simulink library "xrbsComm_r4"  (Simulink 7.1)
PreLoadFcn:
  | warning('off','MATLAB:mex:deprecatedExtension');xlmeta;com.xilinx.sysgen.util.StrategyUtil.loadAllStrategyNames();
undefined symbols (not defined in the file or in its folder): calc_path_data, gcbh, mfcm_matrix_rom, oct2dec, xlBlockLoadCallback
libraries: xbsIndex_r4 x851, mfcm_block_lib_v1 x5, xrbsComm_r4 x1, mfcm_misc_lib_v1 x1
(part 5 of 8)

== system xrbsComm_r4/White Gaussian  Noise Generator/Box-Muller2/fr1/lfsr_41_2/x6 ==
  " " : Inport  OutDataType=sfix(16)  OutScaling=2^0
  reset : Inport  Port=2  OutDataType=sfix(16)  OutScaling=2^0
  ASR : Subsystem  mask{init=[init(8) init(7) init(6) init(5) init(4) init(3) init(2) init(1)]}
      mask prompts: init "Initial Value"
      mask init:
      | init_size = size(init);
      | asr_length = init_size(2);
  Register1 : xbsIndex_r4/Register  init=init(9)  rst=on  en=off  dbl_ovrd=off  block_type=register
      settings: xl_area=[0, 0, 0, 0, 0, 0, 0]  block_version=VER_STRING_GOES_HERE
  z-9 : Outport  OutDataType=sfix(16)  OutScaling=2^0
  wires:
  ASR/1(dout) -> z-9/1
  " "/1 -> Register1/1
  Register1/1 -> ASR/1(din)
  reset/1 -> Register1/2

== system xrbsComm_r4/White Gaussian  Noise Generator/Box-Muller2/fr1/lfsr_41_2/x7 ==
  " " : Inport  OutDataType=sfix(16)  OutScaling=2^0
  reset : Inport  Port=2  OutDataType=sfix(16)  OutScaling=2^0
  ASR : Subsystem  mask{init=[init(8) init(7) init(6) init(5) init(4) init(3) init(2) init(1)]}
      mask prompts: init "Initial Value"
      mask init:
      | init_size = size(init);
      | asr_length = init_size(2);
  Register1 : xbsIndex_r4/Register  init=init(9)  rst=on  en=off  dbl_ovrd=off  block_type=register
      settings: xl_area=[0, 0, 0, 0, 0, 0, 0]  block_version=VER_STRING_GOES_HERE
  z-9 : Outport  OutDataType=sfix(16)  OutScaling=2^0
  wires:
  ASR/1(dout) -> z-9/1
  Register1/1 -> ASR/1(din)
  " "/1 -> Register1/1
  reset/1 -> Register1/2

== system xrbsComm_r4/White Gaussian  Noise Generator/Box-Muller2/g2/lfsr_47_5/x10 ==
  "  " : Inport  OutDataType=sfix(16)  OutScaling=2^0
  reset : Inport  Port=2  OutDataType=sfix(16)  OutScaling=2^0
  ASR : Subsystem  mask{init=[init(4) init(3) init(2) init(1)]}
      mask prompts: init "Initial Value"
      mask init:
      | init_size = size(init);
      | asr_length = init_size(2);
  Register5 : xbsIndex_r4/Register  init=init(5)  rst=on  en=off  dbl_ovrd=off  block_type=register
      settings: xl_area=[0, 0, 0, 0, 0, 0, 0]  block_version=VER_STRING_GOES_HERE
  z-5 : Outport  OutDataType=sfix(16)  OutScaling=2^0
  wires:
  ASR/1(dout) -> z-5/1
  Register5/1 -> ASR/1(din)
  "  "/1 -> Register5/1
  reset/1 -> Register5/2

== system xrbsComm_r4/White Gaussian  Noise Generator/Box-Muller2/g2/lfsr_47_5/x11 ==
  " " : Inport  OutDataType=sfix(16)  OutScaling=2^0
  reset : Inport  Port=2  OutDataType=sfix(16)  OutScaling=2^0
  ASR : Subsystem  mask{init=[init(4) init(3) init(2) init(1)]}
      mask prompts: init "Initial Value"
      mask init:
      | init_size = size(init);
      | asr_length = init_size(2);
  Register : xbsIndex_r4/Register  init=init(5)  rst=on  en=off  dbl_ovrd=off  block_type=register
      settings: xl_area=[0, 0, 0, 0, 0, 0, 0]  block_version=VER_STRING_GOES_HERE
  z-5 : Outport  OutDataType=sfix(16)  OutScaling=2^0
  wires:
  ASR/1(dout) -> z-5/1
  Register/1 -> ASR/1(din)
  " "/1 -> Register/1
  reset/1 -> Register/2

== system xrbsComm_r4/White Gaussian  Noise Generator/Box-Muller2/g2/lfsr_47_5/x12 ==
  " " : Inport  OutDataType=sfix(16)  OutScaling=2^0
  reset : Inport  Port=2  OutDataType=sfix(16)  OutScaling=2^0
  ASR : Subsystem  mask{init=[init(4) init(3) init(2) init(1)]}
      mask prompts: init "Initial Value"
      mask init:
      | init_size = size(init);
      | asr_length = init_size(2);
  Register : xbsIndex_r4/Register  init=init(5)  rst=on  en=off  dbl_ovrd=off  block_type=register
      settings: xl_area=[0, 0, 0, 0, 0, 0, 0]  block_version=VER_STRING_GOES_HERE
  z-5 : Outport  OutDataType=sfix(16)  OutScaling=2^0
  wires:
  ASR/1(dout) -> z-5/1
  Register/1 -> ASR/1(din)
  " "/1 -> Register/1
  reset/1 -> Register/2

== system xrbsComm_r4/White Gaussian  Noise Generator/Box-Muller2/g2/lfsr_47_5/x13 ==
  note: reset
  " " : Inport  OutDataType=sfix(16)  OutScaling=2^0
  " 1" : Inport  Port=2  OutDataType=sfix(16)  OutScaling=2^0
  ASR : Subsystem  mask{init=[init(4) init(3) init(2) init(1)]}
      mask prompts: init "Initial Value"
      mask init:
      | init_size = size(init);
      | asr_length = init_size(2);
  Register : xbsIndex_r4/Register  init=init(5)  rst=on  en=off  dbl_ovrd=off  block_type=register
      settings: xl_area=[0, 0, 0, 0, 0, 0, 0]  block_version=VER_STRING_GOES_HERE
  z-5 : Outport  OutDataType=sfix(16)  OutScaling=2^0
  wires:
  ASR/1(dout) -> z-5/1
  Register/1 -> ASR/1(din)
  " "/1 -> Register/1
  " 1"/1 -> Register/2

== system xrbsComm_r4/White Gaussian  Noise Generator/Box-Muller2/g2/lfsr_47_5/x14 ==
  " " : Inport  OutDataType=sfix(16)  OutScaling=2^0
  reset : Inport  Port=2  OutDataType=sfix(16)  OutScaling=2^0
  ASR : Subsystem  mask{init=[init(4) init(3) init(2) init(1)]}
      mask prompts: init "Initial Value"
      mask init:
      | init_size = size(init);
      | asr_length = init_size(2);
  Register : xbsIndex_r4/Register  init=init(5)  rst=on  en=off  dbl_ovrd=off  block_type=register
      settings: xl_area=[0, 0, 0, 0, 0, 0, 0]  block_version=VER_STRING_GOES_HERE
  z-5 : Outport  OutDataType=sfix(16)  OutScaling=2^0
  wires:
  ASR/1(dout) -> z-5/1
  Register/1 -> ASR/1(din)
  " "/1 -> Register/1
  reset/1 -> Register/2

== system xrbsComm_r4/White Gaussian  Noise Generator/Box-Muller2/g2/lfsr_47_5/x15 ==
  " " : Inport  OutDataType=sfix(16)  OutScaling=2^0
  reset : Inport  Port=2  OutDataType=sfix(16)  OutScaling=2^0
  ASR : Subsystem  mask{init=[init(4) init(3) init(2) init(1)]}
      mask prompts: init "Initial Value"
      mask init:
      | init_size = size(init);
      | asr_length = init_size(2);
  Register : xbsIndex_r4/Register  init=init(5)  rst=on  en=off  dbl_ovrd=off  block_type=register
      settings: xl_area=[0, 0, 0, 0, 0, 0, 0]  block_version=VER_STRING_GOES_HERE
  z-5 : Outport  OutDataType=sfix(16)  OutScaling=2^0
  wires:
  ASR/1(dout) -> z-5/1
  Register/1 -> ASR/1(din)
  " "/1 -> Register/1
  reset/1 -> Register/2

== system xrbsComm_r4/White Gaussian  Noise Generator/Box-Muller2/g2/lfsr_47_5/x16 ==
  " " : Inport  OutDataType=sfix(16)  OutScaling=2^0
  reset : Inport  Port=2  OutDataType=sfix(16)  OutScaling=2^0
  ASR : Subsystem  mask{init=[init(3) init(2) init(1)]}
      mask prompts: init "Initial Value"
      mask init:
      | init_size = size(init);
      | asr_length = init_size(2);
  Register : xbsIndex_r4/Register  init=init(4)  rst=on  en=off  dbl_ovrd=off  block_type=register
      settings: xl_area=[0, 0, 0, 0, 0, 0, 0]  block_version=VER_STRING_GOES_HERE
  z-4 : Outport  OutDataType=sfix(16)  OutScaling=2^0
  wires:
  ASR/1(dout) -> z-4/1
  Register/1 -> ASR/1(din)
  " "/1 -> Register/1
  reset/1 -> Register/2

== system xrbsComm_r4/White Gaussian  Noise Generator/Box-Muller2/g2/lfsr_47_5/x9 ==
  " " : Inport  OutDataType=sfix(16)  OutScaling=2^0
  reset : Inport  Port=2  OutDataType=sfix(16)  OutScaling=2^0
  ASR : Subsystem  mask{init=[init(4) init(3) init(2) init(1)]}
      mask prompts: init "Initial Value"
      mask init:
      | init_size = size(init);
      | asr_length = init_size(2);
  Register : xbsIndex_r4/Register  init=init(5)  rst=on  en=off  dbl_ovrd=off  block_type=register
      settings: xl_area=[0, 0, 0, 0, 0, 0, 0]  block_version=VER_STRING_GOES_HERE
  z-5 : Outport  OutDataType=sfix(16)  OutScaling=2^0
  wires:
  ASR/1(dout) -> z-5/1
  Register/1 -> ASR/1(din)
  " "/1 -> Register/1
  reset/1 -> Register/2

== system xrbsComm_r4/White Gaussian  Noise Generator/Box-Muller3/fr1/lfsr_17_2/x1 ==
  " " : Inport  OutDataType=sfix(16)  OutScaling=2^0
  " reset" : Inport  Port=2  OutDataType=sfix(16)  OutScaling=2^0
  ASR : Subsystem  mask{init=[init(2) init(1)]}
      mask prompts: init "Initial Value"
      mask init:
      | init_size = size(init);
      | asr_length = init_size(2);
  Register4 : xbsIndex_r4/Register  init=init(3)  rst=on  en=off  dbl_ovrd=off  block_type=register
      settings: xl_area=[0, 0, 0, 0, 0, 0, 0]  block_version=VER_STRING_GOES_HERE
  z-3 : Outport  OutDataType=sfix(16)  OutScaling=2^0
  wires:
  " "/1 -> Register4/1
  ASR/1(dout) -> z-3/1
  Register4/1 -> ASR/1(din)
  " reset"/1 -> Register4/2

== system xrbsComm_r4/White Gaussian  Noise Generator/Box-Muller3/fr1/lfsr_17_2/x5 ==
  " " : Inport  OutDataType=sfix(16)  OutScaling=2^0
  reset : Inport  Port=2  OutDataType=sfix(16)  OutScaling=2^0
  ASR : Subsystem  mask{init=[init(3) init(2) init(1)]}
      mask prompts: init "Initial Value"
      mask init:
      | init_size = size(init);
      | asr_length = init_size(2);
  Register5 : xbsIndex_r4/Register  init=init(4)  rst=on  en=off  dbl_ovrd=off  block_type=register
      settings: xl_area=[0, 0, 0, 0, 0, 0, 0]  block_version=VER_STRING_GOES_HERE
  z-4 : Outport  OutDataType=sfix(16)  OutScaling=2^0
  wires:
  ASR/1(dout) -> z-4/1
  Register5/1 -> ASR/1(din)
  " "/1 -> Register5/1
  reset/1 -> Register5/2

== system xrbsComm_r4/White Gaussian  Noise Generator/Box-Muller3/fr1/lfsr_17_2/x6 ==
  " " : Inport  OutDataType=sfix(16)  OutScaling=2^0
  " reset" : Inport  Port=2  OutDataType=sfix(16)  OutScaling=2^0
  ASR : Subsystem  mask{init=[init(2) init(1)]}
      mask prompts: init "Initial Value"
      mask init:
      | init_size = size(init);
      | asr_length = init_size(2);
  Register4 : xbsIndex_r4/Register  init=init(3)  rst=on  en=off  dbl_ovrd=off  block_type=register
      settings: xl_area=[0, 0, 0, 0, 0, 0, 0]  block_version=VER_STRING_GOES_HERE
  z-3 : Outport  OutDataType=sfix(16)  OutScaling=2^0
  wires:
  ASR/1(dout) -> z-3/1
  " "/1 -> Register4/1
  Register4/1 -> ASR/1(din)
  " reset"/1 -> Register4/2

== system xrbsComm_r4/White Gaussian  Noise Generator/Box-Muller3/fr1/lfsr_17_2/x7 ==
  " " : Inport  OutDataType=sfix(16)  OutScaling=2^0
  reset : Inport  Port=2  OutDataType=sfix(16)  OutScaling=2^0
  ASR : Subsystem  mask{init=[init(2) init(1)]}
      mask prompts: init "Initial Value"
      mask init:
      | init_size = size(init);
      | asr_length = init_size(2);
  Register4 : xbsIndex_r4/Register  init=init(3)  rst=on  en=off  dbl_ovrd=off  block_type=register
      settings: xl_area=[0, 0, 0, 0, 0, 0, 0]  block_version=VER_STRING_GOES_HERE
  z-3 : Outport  OutDataType=sfix(16)  OutScaling=2^0
  wires:
  " "/1 -> Register4/1
  ASR/1(dout) -> z-3/1
  Register4/1 -> ASR/1(din)
  reset/1 -> Register4/2

== system xrbsComm_r4/White Gaussian  Noise Generator/Box-Muller3/fr1/lfsr_25_2/x1 ==
  " " : Inport  OutDataType=sfix(16)  OutScaling=2^0
  reset : Inport  Port=2  OutDataType=sfix(16)  OutScaling=2^0
  ASR : Subsystem  mask{init=[init(4) init(3) init(2) init(1)]}
      mask prompts: init "Initial Value"
      mask init:
      | init_size = size(init);
      | asr_length = init_size(2);
  Register : xbsIndex_r4/Register  init=init(5)  rst=on  en=off  dbl_ovrd=off  block_type=register
      settings: xl_area=[0, 0, 0, 0, 0, 0, 0]  block_version=VER_STRING_GOES_HERE
  z-5 : Outport  OutDataType=sfix(16)  OutScaling=2^0
  wires:
  Register/1 -> ASR/1(din)
  ASR/1(dout) -> z-5/1
  " "/1 -> Register/1
  reset/1 -> Register/2

== system xrbsComm_r4/White Gaussian  Noise Generator/Box-Muller3/fr1/lfsr_25_2/x5 ==
  " " : Inport  OutDataType=sfix(16)  OutScaling=2^0
  reset : Inport  Port=2  OutDataType=sfix(16)  OutScaling=2^0
  ASR : Subsystem  mask{init=[init(5) init(4) init(3) init(2) init(1)]}
      mask prompts: init "Initial Value"
      mask init:
      | init_size = size(init);
      | asr_length = init_size(2);
  Register : xbsIndex_r4/Register  init=init(6)  rst=on  en=off  dbl_ovrd=off  block_type=register
      settings: xl_area=[0, 0, 0, 0, 0, 0, 0]  block_version=VER_STRING_GOES_HERE
  z-6 : Outport  OutDataType=sfix(16)  OutScaling=2^0
  wires:
  Register/1 -> ASR/1(din)
  ASR/1(dout) -> z-6/1
  " "/1 -> Register/1
  reset/1 -> Register/2

== system xrbsComm_r4/White Gaussian  Noise Generator/Box-Muller3/fr1/lfsr_25_2/x6 ==
  " " : Inport  OutDataType=sfix(16)  OutScaling=2^0
  reset : Inport  Port=2  OutDataType=sfix(16)  OutScaling=2^0
  ASR : Subsystem  mask{init=[init(4) init(3) init(2) init(1)]}
      mask prompts: init "Initial Value"
      mask init:
      | init_size = size(init);
      | asr_length = init_size(2);
  Register : xbsIndex_r4/Register  init=init(5)  rst=on  en=off  dbl_ovrd=off  block_type=register
      settings: xl_area=[0, 0, 0, 0, 0, 0, 0]  block_version=VER_STRING_GOES_HERE
  z-5 : Outport  OutDataType=sfix(16)  OutScaling=2^0
  wires:
  Register/1 -> ASR/1(din)
  ASR/1(dout) -> z-5/1
  " "/1 -> Register/1
  reset/1 -> Register/2

== system xrbsComm_r4/White Gaussian  Noise Generator/Box-Muller3/fr1/lfsr_25_2/x7 ==
  " " : Inport  OutDataType=sfix(16)  OutScaling=2^0
  reset : Inport  Port=2  OutDataType=sfix(16)  OutScaling=2^0
  ASR : Subsystem  mask{init=[init(4) init(3) init(2) init(1)]}
      mask prompts: init "Initial Value"
      mask init:
      | init_size = size(init);
      | asr_length = init_size(2);
  Register : xbsIndex_r4/Register  init=init(5)  rst=on  en=off  dbl_ovrd=off  block_type=register
      settings: xl_area=[0, 0, 0, 0, 0, 0, 0]  block_version=VER_STRING_GOES_HERE
  z-5 : Outport  OutDataType=sfix(16)  OutScaling=2^0
  wires:
  Register/1 -> ASR/1(din)
  ASR/1(dout) -> z-5/1
  " "/1 -> Register/1
  reset/1 -> Register/2

== system xrbsComm_r4/White Gaussian  Noise Generator/Box-Muller3/fr1/lfsr_29_2/x5 ==
  " " : Inport  OutDataType=sfix(16)  OutScaling=2^0
  reset : Inport  Port=2  OutDataType=sfix(16)  OutScaling=2^0
  ASR : Subsystem  mask{init=[init(6) init(5) init(4) init(3) init(2) init(1)]}
      mask prompts: init "Initial Value"
      mask init:
      | init_size = size(init);
      | asr_length = init_size(2);
  Register : xbsIndex_r4/Register  init=init(7)  rst=on  en=off  dbl_ovrd=off  block_type=register
      settings: xl_area=[0, 0, 0, 0, 0, 0, 0]  block_version=VER_STRING_GOES_HERE
  z-7 : Outport  OutDataType=sfix(16)  OutScaling=2^0
  wires:
  ASR/1(dout) -> z-7/1
  Register/1 -> ASR/1(din)
  " "/1 -> Register/1
  reset/1 -> Register/2

== system xrbsComm_r4/White Gaussian  Noise Generator/Box-Muller3/fr1/lfsr_29_2/x6 ==
  " " : Inport  OutDataType=sfix(16)  OutScaling=2^0
  reset : Inport  Port=2  OutDataType=sfix(16)  OutScaling=2^0
  ASR : Subsystem  mask{init=[init(5) init(4) init(3) init(2) init(1)]}
      mask prompts: init "Initial Value"
      mask init:
      | init_size = size(init);
      | asr_length = init_size(2);
  Register : xbsIndex_r4/Register  init=init(6)  rst=on  en=off  dbl_ovrd=off  block_type=register
      settings: xl_area=[0, 0, 0, 0, 0, 0, 0]  block_version=VER_STRING_GOES_HERE
  z-6 : Outport  OutDataType=sfix(16)  OutScaling=2^0
  wires:
  ASR/1(dout) -> z-6/1
  Register/1 -> ASR/1(din)
  " "/1 -> Register/1
  reset/1 -> Register/2

== system xrbsComm_r4/White Gaussian  Noise Generator/Box-Muller3/fr1/lfsr_29_2/x7 ==
  " " : Inport  OutDataType=sfix(16)  OutScaling=2^0
  reset : Inport  Port=2  OutDataType=sfix(16)  OutScaling=2^0
  ASR : Subsystem  mask{init=[init(5) init(4) init(3) init(2) init(1)]}
      mask prompts: init "Initial Value"
      mask init:
      | init_size = size(init);
      | asr_length = init_size(2);
  Register : xbsIndex_r4/Register  init=init(6)  rst=on  en=off  dbl_ovrd=off  block_type=register
      settings: xl_area=[0, 0, 0, 0, 0, 0, 0]  block_version=VER_STRING_GOES_HERE
  z-6 : Outport  OutDataType=sfix(16)  OutScaling=2^0
  wires:
  ASR/1(dout) -> z-6/1
  Register/1 -> ASR/1(din)
  " "/1 -> Register/1
  reset/1 -> Register/2

== system xrbsComm_r4/White Gaussian  Noise Generator/Box-Muller3/fr1/lfsr_29_2/x8 ==
  " " : Inport  OutDataType=sfix(16)  OutScaling=2^0
  reset : Inport  Port=2  OutDataType=sfix(16)  OutScaling=2^0
  ASR : Subsystem  mask{init=[init(5) init(4) init(3) init(2) init(1)]}
      mask prompts: init "Initial Value"
      mask init:
      | init_size = size(init);
      | asr_length = init_size(2);
  Register : xbsIndex_r4/Register  init=init(6)  rst=on  en=off  dbl_ovrd=off  block_type=register
      settings: xl_area=[0, 0, 0, 0, 0, 0, 0]  block_version=VER_STRING_GOES_HERE
  z-6 : Outport  OutDataType=sfix(16)  OutScaling=2^0
  wires:
  ASR/1(dout) -> z-6/1
  Register/1 -> ASR/1(din)
  " "/1 -> Register/1
  reset/1 -> Register/2

== system xrbsComm_r4/White Gaussian  Noise Generator/Box-Muller3/fr1/lfsr_31_2/x5 ==
  " " : Inport  OutDataType=sfix(16)  OutScaling=2^0
  reset : Inport  Port=2  OutDataType=sfix(16)  OutScaling=2^0
  ASR : Subsystem  mask{init=[init(6) init(5) init(4) init(3) init(2) init(1)]}
      mask prompts: init "Initial Value"
      mask init:
      | init_size = size(init);
      | asr_length = init_size(2);
  Register : xbsIndex_r4/Register  init=init(7)  rst=on  en=off  dbl_ovrd=off  block_type=register
      settings: xl_area=[0, 0, 0, 0, 0, 0, 0]  block_version=VER_STRING_GOES_HERE
  z-7 : Outport  OutDataType=sfix(16)  OutScaling=2^0
  wires:
  Register/1 -> ASR/1(din)
  ASR/1(dout) -> z-7/1
  " "/1 -> Register/1
  reset/1 -> Register/2

== system xrbsComm_r4/White Gaussian  Noise Generator/Box-Muller3/fr1/lfsr_31_2/x6 ==
  " " : Inport  OutDataType=sfix(16)  OutScaling=2^0
  reset : Inport  Port=2  OutDataType=sfix(16)  OutScaling=2^0
  ASR : Subsystem  mask{init=[init(6) init(5) init(4) init(3) init(2) init(1)]}
      mask prompts: init "Initial Value"
      mask init:
      | init_size = size(init);
      | asr_length = init_size(2);
  Register : xbsIndex_r4/Register  init=init(7)  rst=on  en=off  dbl_ovrd=off  block_type=register
      settings: xl_area=[0, 0, 0, 0, 0, 0, 0]  block_version=VER_STRING_GOES_HERE
  z-7 : Outport  OutDataType=sfix(16)  OutScaling=2^0
  wires:
  Register/1 -> ASR/1(din)
  " "/1 -> Register/1
  ASR/1(dout) -> z-7/1
  reset/1 -> Register/2

== system xrbsComm_r4/White Gaussian  Noise Generator/Box-Muller3/fr1/lfsr_31_2/x7 ==
  " " : Inport  OutDataType=sfix(16)  OutScaling=2^0
  reset : Inport  Port=2  OutDataType=sfix(16)  OutScaling=2^0
  ASR : Subsystem  mask{init=[init(6) init(5) init(4) init(3) init(2) init(1)]}
      mask prompts: init "Initial Value"
      mask init:
      | init_size = size(init);
      | asr_length = init_size(2);
  Register : xbsIndex_r4/Register  init=init(7)  rst=on  en=off  dbl_ovrd=off  block_type=register
      settings: xl_area=[0, 0, 0, 0, 0, 0, 0]  block_version=VER_STRING_GOES_HERE
  z-7 : Outport  OutDataType=sfix(16)  OutScaling=2^0
  wires:
  Register/1 -> ASR/1(din)
  ASR/1(dout) -> z-7/1
  " "/1 -> Register/1
  reset/1 -> Register/2

== system xrbsComm_r4/White Gaussian  Noise Generator/Box-Muller3/fr1/lfsr_31_2/x8 ==
  " " : Inport  OutDataType=sfix(16)  OutScaling=2^0
  reset : Inport  Port=2  OutDataType=sfix(16)  OutScaling=2^0
  ASR : Subsystem  mask{init=[init(5) init(4) init(3) init(2) init(1)]}
      mask prompts: init "Initial Value"
      mask init:
      | init_size = size(init);
      | asr_length = init_size(2);
  Register : xbsIndex_r4/Register  init=init(6)  rst=on  en=off  dbl_ovrd=off  block_type=register
      settings: xl_area=[0, 0, 0, 0, 0, 0, 0]  block_version=VER_STRING_GOES_HERE
  z-6 : Outport  OutDataType=sfix(16)  OutScaling=2^0
  wires:
  Register/1 -> ASR/1(din)
  " "/1 -> Register/1
  ASR/1(dout) -> z-6/1
  reset/1 -> Register/2

== system xrbsComm_r4/White Gaussian  Noise Generator/Box-Muller3/fr1/lfsr_41_2/x1 ==
  " " : Inport  OutDataType=sfix(16)  OutScaling=2^0
  reset : Inport  Port=2  OutDataType=sfix(16)  OutScaling=2^0
  ASR : Subsystem  mask{init=[init(8) init(7) init(6) init(5) init(4) init(3) init(2) init(1)]}
      mask prompts: init "Initial Value"
      mask init:
      | init_size = size(init);
      | asr_length = init_size(2);
  Register1 : xbsIndex_r4/Register  init=init(9)  rst=on  en=off  dbl_ovrd=off  block_type=register
      settings: xl_area=[0, 0, 0, 0, 0, 0, 0]  block_version=VER_STRING_GOES_HERE
  z-9 : Outport  OutDataType=sfix(16)  OutScaling=2^0
  wires:
  ASR/1(dout) -> z-9/1
  " "/1 -> Register1/1
  Register1/1 -> ASR/1(din)
  reset/1 -> Register1/2

== system xrbsComm_r4/White Gaussian  Noise Generator/Box-Muller3/fr1/lfsr_41_2/x5 ==
  " " : Inport  OutDataType=sfix(16)  OutScaling=2^0
  reset : Inport  Port=2  OutDataType=sfix(16)  OutScaling=2^0
  ASR : Subsystem  mask{init=[init(9) init(8) init(7) init(6) init(5) init(4) init(3) init(2) init(1)]}
      mask prompts: init "Initial Value"
      mask init:
      | init_size = size(init);
      | asr_length = init_size(2);
  Register : xbsIndex_r4/Register  init=init(10)  rst=on  en=off  dbl_ovrd=off  block_type=register
      settings: xl_area=[0, 0, 0, 0, 0, 0, 0]  block_version=VER_STRING_GOES_HERE
  z-10 : Outport  OutDataType=sfix(16)  OutScaling=2^0
  wires:
  Register/1 -> ASR/1(din)
  ASR/1(dout) -> z-10/1
  " "/1 -> Register/1
  reset/1 -> Register/2

== system xrbsComm_r4/White Gaussian  Noise Generator/Box-Muller3/fr1/lfsr_41_2/x6 ==
  " " : Inport  OutDataType=sfix(16)  OutScaling=2^0
  reset : Inport  Port=2  OutDataType=sfix(16)  OutScaling=2^0
  ASR : Subsystem  mask{init=[init(8) init(7) init(6) init(5) init(4) init(3) init(2) init(1)]}
      mask prompts: init "Initial Value"
      mask init:
      | init_size = size(init);
      | asr_length = init_size(2);
  Register1 : xbsIndex_r4/Register  init=init(9)  rst=on  en=off  dbl_ovrd=off  block_type=register
      settings: xl_area=[0, 0, 0, 0, 0, 0, 0]  block_version=VER_STRING_GOES_HERE
  z-9 : Outport  OutDataType=sfix(16)  OutScaling=2^0
  wires:
  ASR/1(dout) -> z-9/1
  " "/1 -> Register1/1
  Register1/1 -> ASR/1(din)
  reset/1 -> Register1/2

== system xrbsComm_r4/White Gaussian  Noise Generator/Box-Muller3/fr1/lfsr_41_2/x7 ==
  " " : Inport  OutDataType=sfix(16)  OutScaling=2^0
  reset : Inport  Port=2  OutDataType=sfix(16)  OutScaling=2^0
  ASR : Subsystem  mask{init=[init(8) init(7) init(6) init(5) init(4) init(3) init(2) init(1)]}
      mask prompts: init "Initial Value"
      mask init:
      | init_size = size(init);
      | asr_length = init_size(2);
  Register1 : xbsIndex_r4/Register  init=init(9)  rst=on  en=off  dbl_ovrd=off  block_type=register
      settings: xl_area=[0, 0, 0, 0, 0, 0, 0]  block_version=VER_STRING_GOES_HERE
  z-9 : Outport  OutDataType=sfix(16)  OutScaling=2^0
  wires:
  ASR/1(dout) -> z-9/1
  Register1/1 -> ASR/1(din)
  " "/1 -> Register1/1
  reset/1 -> Register1/2

== system xrbsComm_r4/White Gaussian  Noise Generator/Box-Muller3/g2/lfsr_47_5/x10 ==
  "  " : Inport  OutDataType=sfix(16)  OutScaling=2^0
  reset : Inport  Port=2  OutDataType=sfix(16)  OutScaling=2^0
  ASR : Subsystem  mask{init=[init(4) init(3) init(2) init(1)]}
      mask prompts: init "Initial Value"
      mask init:
      | init_size = size(init);
      | asr_length = init_size(2);
  Register5 : xbsIndex_r4/Register  init=init(5)  rst=on  en=off  dbl_ovrd=off  block_type=register
      settings: xl_area=[0, 0, 0, 0, 0, 0, 0]  block_version=VER_STRING_GOES_HERE
  z-5 : Outport  OutDataType=sfix(16)  OutScaling=2^0
  wires:
  ASR/1(dout) -> z-5/1
  Register5/1 -> ASR/1(din)
  "  "/1 -> Register5/1
  reset/1 -> Register5/2

== system xrbsComm_r4/White Gaussian  Noise Generator/Box-Muller3/g2/lfsr_47_5/x11 ==
  " " : Inport  OutDataType=sfix(16)  OutScaling=2^0
  reset : Inport  Port=2  OutDataType=sfix(16)  OutScaling=2^0
  ASR : Subsystem  mask{init=[init(4) init(3) init(2) init(1)]}
      mask prompts: init "Initial Value"
      mask init:
      | init_size = size(init);
      | asr_length = init_size(2);
  Register : xbsIndex_r4/Register  init=init(5)  rst=on  en=off  dbl_ovrd=off  block_type=register
      settings: xl_area=[0, 0, 0, 0, 0, 0, 0]  block_version=VER_STRING_GOES_HERE
  z-5 : Outport  OutDataType=sfix(16)  OutScaling=2^0
  wires:
  ASR/1(dout) -> z-5/1
  Register/1 -> ASR/1(din)
  " "/1 -> Register/1
  reset/1 -> Register/2

== system xrbsComm_r4/White Gaussian  Noise Generator/Box-Muller3/g2/lfsr_47_5/x12 ==
  " " : Inport  OutDataType=sfix(16)  OutScaling=2^0
  reset : Inport  Port=2  OutDataType=sfix(16)  OutScaling=2^0
  ASR : Subsystem  mask{init=[init(4) init(3) init(2) init(1)]}
      mask prompts: init "Initial Value"
      mask init:
      | init_size = size(init);
      | asr_length = init_size(2);
  Register : xbsIndex_r4/Register  init=init(5)  rst=on  en=off  dbl_ovrd=off  block_type=register
      settings: xl_area=[0, 0, 0, 0, 0, 0, 0]  block_version=VER_STRING_GOES_HERE
  z-5 : Outport  OutDataType=sfix(16)  OutScaling=2^0
  wires:
  ASR/1(dout) -> z-5/1
  Register/1 -> ASR/1(din)
  " "/1 -> Register/1
  reset/1 -> Register/2

== system xrbsComm_r4/White Gaussian  Noise Generator/Box-Muller3/g2/lfsr_47_5/x13 ==
  note: reset
  " " : Inport  OutDataType=sfix(16)  OutScaling=2^0
  " 1" : Inport  Port=2  OutDataType=sfix(16)  OutScaling=2^0
  ASR : Subsystem  mask{init=[init(4) init(3) init(2) init(1)]}
      mask prompts: init "Initial Value"
      mask init:
      | init_size = size(init);
      | asr_length = init_size(2);
  Register : xbsIndex_r4/Register  init=init(5)  rst=on  en=off  dbl_ovrd=off  block_type=register
      settings: xl_area=[0, 0, 0, 0, 0, 0, 0]  block_version=VER_STRING_GOES_HERE
  z-5 : Outport  OutDataType=sfix(16)  OutScaling=2^0
  wires:
  ASR/1(dout) -> z-5/1
  Register/1 -> ASR/1(din)
  " "/1 -> Register/1
  " 1"/1 -> Register/2

== system xrbsComm_r4/White Gaussian  Noise Generator/Box-Muller3/g2/lfsr_47_5/x14 ==
  " " : Inport  OutDataType=sfix(16)  OutScaling=2^0
  reset : Inport  Port=2  OutDataType=sfix(16)  OutScaling=2^0
  ASR : Subsystem  mask{init=[init(4) init(3) init(2) init(1)]}
      mask prompts: init "Initial Value"
      mask init:
      | init_size = size(init);
      | asr_length = init_size(2);
  Register : xbsIndex_r4/Register  init=init(5)  rst=on  en=off  dbl_ovrd=off  block_type=register
      settings: xl_area=[0, 0, 0, 0, 0, 0, 0]  block_version=VER_STRING_GOES_HERE
  z-5 : Outport  OutDataType=sfix(16)  OutScaling=2^0
  wires:
  ASR/1(dout) -> z-5/1
  Register/1 -> ASR/1(din)
  " "/1 -> Register/1
  reset/1 -> Register/2

== system xrbsComm_r4/White Gaussian  Noise Generator/Box-Muller3/g2/lfsr_47_5/x15 ==
  " " : Inport  OutDataType=sfix(16)  OutScaling=2^0
  reset : Inport  Port=2  OutDataType=sfix(16)  OutScaling=2^0
  ASR : Subsystem  mask{init=[init(4) init(3) init(2) init(1)]}
      mask prompts: init "Initial Value"
      mask init:
      | init_size = size(init);
      | asr_length = init_size(2);
  Register : xbsIndex_r4/Register  init=init(5)  rst=on  en=off  dbl_ovrd=off  block_type=register
      settings: xl_area=[0, 0, 0, 0, 0, 0, 0]  block_version=VER_STRING_GOES_HERE
  z-5 : Outport  OutDataType=sfix(16)  OutScaling=2^0
  wires:
  ASR/1(dout) -> z-5/1
  Register/1 -> ASR/1(din)
  " "/1 -> Register/1
  reset/1 -> Register/2

== system xrbsComm_r4/White Gaussian  Noise Generator/Box-Muller3/g2/lfsr_47_5/x16 ==
  " " : Inport  OutDataType=sfix(16)  OutScaling=2^0
  reset : Inport  Port=2  OutDataType=sfix(16)  OutScaling=2^0
  ASR : Subsystem  mask{init=[init(3) init(2) init(1)]}
      mask prompts: init "Initial Value"
      mask init:
      | init_size = size(init);
      | asr_length = init_size(2);
  Register : xbsIndex_r4/Register  init=init(4)  rst=on  en=off  dbl_ovrd=off  block_type=register
      settings: xl_area=[0, 0, 0, 0, 0, 0, 0]  block_version=VER_STRING_GOES_HERE
  z-4 : Outport  OutDataType=sfix(16)  OutScaling=2^0
  wires:
  ASR/1(dout) -> z-4/1
  Register/1 -> ASR/1(din)
  " "/1 -> Register/1
  reset/1 -> Register/2

== system xrbsComm_r4/White Gaussian  Noise Generator/Box-Muller3/g2/lfsr_47_5/x9 ==
  " " : Inport  OutDataType=sfix(16)  OutScaling=2^0
  reset : Inport  Port=2  OutDataType=sfix(16)  OutScaling=2^0
  ASR : Subsystem  mask{init=[init(4) init(3) init(2) init(1)]}
      mask prompts: init "Initial Value"
      mask init:
      | init_size = size(init);
      | asr_length = init_size(2);
  Register : xbsIndex_r4/Register  init=init(5)  rst=on  en=off  dbl_ovrd=off  block_type=register
      settings: xl_area=[0, 0, 0, 0, 0, 0, 0]  block_version=VER_STRING_GOES_HERE
  z-5 : Outport  OutDataType=sfix(16)  OutScaling=2^0
  wires:
  ASR/1(dout) -> z-5/1
  Register/1 -> ASR/1(din)
  " "/1 -> Register/1
  reset/1 -> Register/2

== system xrbsComm_r4/White Gaussian  Noise Generator/Box-Muller4/fr1/lfsr_17_2/x1 ==
  " " : Inport  OutDataType=sfix(16)  OutScaling=2^0
  " reset" : Inport  Port=2  OutDataType=sfix(16)  OutScaling=2^0
  ASR : Subsystem  mask{init=[init(2) init(1)]}
      mask prompts: init "Initial Value"
      mask init:
      | init_size = size(init);
      | asr_length = init_size(2);
  Register4 : xbsIndex_r4/Register  init=init(3)  rst=on  en=off  dbl_ovrd=off  block_type=register
      settings: xl_area=[0, 0, 0, 0, 0, 0, 0]  block_version=VER_STRING_GOES_HERE
  z-3 : Outport  OutDataType=sfix(16)  OutScaling=2^0
  wires:
  " "/1 -> Register4/1
  ASR/1(dout) -> z-3/1
  Register4/1 -> ASR/1(din)
  " reset"/1 -> Register4/2

== system xrbsComm_r4/White Gaussian  Noise Generator/Box-Muller4/fr1/lfsr_17_2/x5 ==
  " " : Inport  OutDataType=sfix(16)  OutScaling=2^0
  reset : Inport  Port=2  OutDataType=sfix(16)  OutScaling=2^0
  ASR : Subsystem  mask{init=[init(3) init(2) init(1)]}
      mask prompts: init "Initial Value"
      mask init:
      | init_size = size(init);
      | asr_length = init_size(2);
  Register5 : xbsIndex_r4/Register  init=init(4)  rst=on  en=off  dbl_ovrd=off  block_type=register
      settings: xl_area=[0, 0, 0, 0, 0, 0, 0]  block_version=VER_STRING_GOES_HERE
  z-4 : Outport  OutDataType=sfix(16)  OutScaling=2^0
  wires:
  ASR/1(dout) -> z-4/1
  Register5/1 -> ASR/1(din)
  " "/1 -> Register5/1
  reset/1 -> Register5/2

== system xrbsComm_r4/White Gaussian  Noise Generator/Box-Muller4/fr1/lfsr_17_2/x6 ==
  " " : Inport  OutDataType=sfix(16)  OutScaling=2^0
  " reset" : Inport  Port=2  OutDataType=sfix(16)  OutScaling=2^0
  ASR : Subsystem  mask{init=[init(2) init(1)]}
      mask prompts: init "Initial Value"
      mask init:
      | init_size = size(init);
      | asr_length = init_size(2);
  Register4 : xbsIndex_r4/Register  init=init(3)  rst=on  en=off  dbl_ovrd=off  block_type=register
      settings: xl_area=[0, 0, 0, 0, 0, 0, 0]  block_version=VER_STRING_GOES_HERE
  z-3 : Outport  OutDataType=sfix(16)  OutScaling=2^0
  wires:
  ASR/1(dout) -> z-3/1
  " "/1 -> Register4/1
  Register4/1 -> ASR/1(din)
  " reset"/1 -> Register4/2

== system xrbsComm_r4/White Gaussian  Noise Generator/Box-Muller4/fr1/lfsr_17_2/x7 ==
  " " : Inport  OutDataType=sfix(16)  OutScaling=2^0
  reset : Inport  Port=2  OutDataType=sfix(16)  OutScaling=2^0
  ASR : Subsystem  mask{init=[init(2) init(1)]}
      mask prompts: init "Initial Value"
      mask init:
      | init_size = size(init);
      | asr_length = init_size(2);
  Register4 : xbsIndex_r4/Register  init=init(3)  rst=on  en=off  dbl_ovrd=off  block_type=register
      settings: xl_area=[0, 0, 0, 0, 0, 0, 0]  block_version=VER_STRING_GOES_HERE
  z-3 : Outport  OutDataType=sfix(16)  OutScaling=2^0
  wires:
  " "/1 -> Register4/1
  ASR/1(dout) -> z-3/1
  Register4/1 -> ASR/1(din)
  reset/1 -> Register4/2

== system xrbsComm_r4/White Gaussian  Noise Generator/Box-Muller4/fr1/lfsr_25_2/x1 ==
  " " : Inport  OutDataType=sfix(16)  OutScaling=2^0
  reset : Inport  Port=2  OutDataType=sfix(16)  OutScaling=2^0
  ASR : Subsystem  mask{init=[init(4) init(3) init(2) init(1)]}
      mask prompts: init "Initial Value"
      mask init:
      | init_size = size(init);
      | asr_length = init_size(2);
  Register : xbsIndex_r4/Register  init=init(5)  rst=on  en=off  dbl_ovrd=off  block_type=register
      settings: xl_area=[0, 0, 0, 0, 0, 0, 0]  block_version=VER_STRING_GOES_HERE
  z-5 : Outport  OutDataType=sfix(16)  OutScaling=2^0
  wires:
  Register/1 -> ASR/1(din)
  ASR/1(dout) -> z-5/1
  " "/1 -> Register/1
  reset/1 -> Register/2

== system xrbsComm_r4/White Gaussian  Noise Generator/Box-Muller4/fr1/lfsr_25_2/x5 ==
  " " : Inport  OutDataType=sfix(16)  OutScaling=2^0
  reset : Inport  Port=2  OutDataType=sfix(16)  OutScaling=2^0
  ASR : Subsystem  mask{init=[init(5) init(4) init(3) init(2) init(1)]}
      mask prompts: init "Initial Value"
      mask init:
      | init_size = size(init);
      | asr_length = init_size(2);
  Register : xbsIndex_r4/Register  init=init(6)  rst=on  en=off  dbl_ovrd=off  block_type=register
      settings: xl_area=[0, 0, 0, 0, 0, 0, 0]  block_version=VER_STRING_GOES_HERE
  z-6 : Outport  OutDataType=sfix(16)  OutScaling=2^0
  wires:
  Register/1 -> ASR/1(din)
  ASR/1(dout) -> z-6/1
  " "/1 -> Register/1
  reset/1 -> Register/2

== system xrbsComm_r4/White Gaussian  Noise Generator/Box-Muller4/fr1/lfsr_25_2/x6 ==
  " " : Inport  OutDataType=sfix(16)  OutScaling=2^0
  reset : Inport  Port=2  OutDataType=sfix(16)  OutScaling=2^0
  ASR : Subsystem  mask{init=[init(4) init(3) init(2) init(1)]}
      mask prompts: init "Initial Value"
      mask init:
      | init_size = size(init);
      | asr_length = init_size(2);
  Register : xbsIndex_r4/Register  init=init(5)  rst=on  en=off  dbl_ovrd=off  block_type=register
      settings: xl_area=[0, 0, 0, 0, 0, 0, 0]  block_version=VER_STRING_GOES_HERE
  z-5 : Outport  OutDataType=sfix(16)  OutScaling=2^0
  wires:
  Register/1 -> ASR/1(din)
  ASR/1(dout) -> z-5/1
  " "/1 -> Register/1
  reset/1 -> Register/2

== system xrbsComm_r4/White Gaussian  Noise Generator/Box-Muller4/fr1/lfsr_25_2/x7 ==
  " " : Inport  OutDataType=sfix(16)  OutScaling=2^0
  reset : Inport  Port=2  OutDataType=sfix(16)  OutScaling=2^0
  ASR : Subsystem  mask{init=[init(4) init(3) init(2) init(1)]}
      mask prompts: init "Initial Value"
      mask init:
      | init_size = size(init);
      | asr_length = init_size(2);
  Register : xbsIndex_r4/Register  init=init(5)  rst=on  en=off  dbl_ovrd=off  block_type=register
      settings: xl_area=[0, 0, 0, 0, 0, 0, 0]  block_version=VER_STRING_GOES_HERE
  z-5 : Outport  OutDataType=sfix(16)  OutScaling=2^0
  wires:
  Register/1 -> ASR/1(din)
  ASR/1(dout) -> z-5/1
  " "/1 -> Register/1
  reset/1 -> Register/2

== system xrbsComm_r4/White Gaussian  Noise Generator/Box-Muller4/fr1/lfsr_29_2/x5 ==
  " " : Inport  OutDataType=sfix(16)  OutScaling=2^0
  reset : Inport  Port=2  OutDataType=sfix(16)  OutScaling=2^0
  ASR : Subsystem  mask{init=[init(6) init(5) init(4) init(3) init(2) init(1)]}
      mask prompts: init "Initial Value"
      mask init:
      | init_size = size(init);
      | asr_length = init_size(2);
  Register : xbsIndex_r4/Register  init=init(7)  rst=on  en=off  dbl_ovrd=off  block_type=register
      settings: xl_area=[0, 0, 0, 0, 0, 0, 0]  block_version=VER_STRING_GOES_HERE
  z-7 : Outport  OutDataType=sfix(16)  OutScaling=2^0
  wires:
  ASR/1(dout) -> z-7/1
  Register/1 -> ASR/1(din)
  " "/1 -> Register/1
  reset/1 -> Register/2

== system xrbsComm_r4/White Gaussian  Noise Generator/Box-Muller4/fr1/lfsr_29_2/x6 ==
  " " : Inport  OutDataType=sfix(16)  OutScaling=2^0
  reset : Inport  Port=2  OutDataType=sfix(16)  OutScaling=2^0
  ASR : Subsystem  mask{init=[init(5) init(4) init(3) init(2) init(1)]}
      mask prompts: init "Initial Value"
      mask init:
      | init_size = size(init);
      | asr_length = init_size(2);
  Register : xbsIndex_r4/Register  init=init(6)  rst=on  en=off  dbl_ovrd=off  block_type=register
      settings: xl_area=[0, 0, 0, 0, 0, 0, 0]  block_version=VER_STRING_GOES_HERE
  z-6 : Outport  OutDataType=sfix(16)  OutScaling=2^0
  wires:
  ASR/1(dout) -> z-6/1
  Register/1 -> ASR/1(din)
  " "/1 -> Register/1
  reset/1 -> Register/2

== system xrbsComm_r4/White Gaussian  Noise Generator/Box-Muller4/fr1/lfsr_29_2/x7 ==
  " " : Inport  OutDataType=sfix(16)  OutScaling=2^0
  reset : Inport  Port=2  OutDataType=sfix(16)  OutScaling=2^0
  ASR : Subsystem  mask{init=[init(5) init(4) init(3) init(2) init(1)]}
      mask prompts: init "Initial Value"
      mask init:
      | init_size = size(init);
      | asr_length = init_size(2);
  Register : xbsIndex_r4/Register  init=init(6)  rst=on  en=off  dbl_ovrd=off  block_type=register
      settings: xl_area=[0, 0, 0, 0, 0, 0, 0]  block_version=VER_STRING_GOES_HERE
  z-6 : Outport  OutDataType=sfix(16)  OutScaling=2^0
  wires:
  ASR/1(dout) -> z-6/1
  Register/1 -> ASR/1(din)
  " "/1 -> Register/1
  reset/1 -> Register/2

== system xrbsComm_r4/White Gaussian  Noise Generator/Box-Muller4/fr1/lfsr_29_2/x8 ==
  " " : Inport  OutDataType=sfix(16)  OutScaling=2^0
  reset : Inport  Port=2  OutDataType=sfix(16)  OutScaling=2^0
  ASR : Subsystem  mask{init=[init(5) init(4) init(3) init(2) init(1)]}
      mask prompts: init "Initial Value"
      mask init:
      | init_size = size(init);
      | asr_length = init_size(2);
  Register : xbsIndex_r4/Register  init=init(6)  rst=on  en=off  dbl_ovrd=off  block_type=register
      settings: xl_area=[0, 0, 0, 0, 0, 0, 0]  block_version=VER_STRING_GOES_HERE
  z-6 : Outport  OutDataType=sfix(16)  OutScaling=2^0
  wires:
  ASR/1(dout) -> z-6/1
  Register/1 -> ASR/1(din)
  " "/1 -> Register/1
  reset/1 -> Register/2

== system xrbsComm_r4/White Gaussian  Noise Generator/Box-Muller4/fr1/lfsr_31_2/x5 ==
  " " : Inport  OutDataType=sfix(16)  OutScaling=2^0
  reset : Inport  Port=2  OutDataType=sfix(16)  OutScaling=2^0
  ASR : Subsystem  mask{init=[init(6) init(5) init(4) init(3) init(2) init(1)]}
      mask prompts: init "Initial Value"
      mask init:
      | init_size = size(init);
      | asr_length = init_size(2);
  Register : xbsIndex_r4/Register  init=init(7)  rst=on  en=off  dbl_ovrd=off  block_type=register
      settings: xl_area=[0, 0, 0, 0, 0, 0, 0]  block_version=VER_STRING_GOES_HERE
  z-7 : Outport  OutDataType=sfix(16)  OutScaling=2^0
  wires:
  Register/1 -> ASR/1(din)
  ASR/1(dout) -> z-7/1
  " "/1 -> Register/1
  reset/1 -> Register/2

== system xrbsComm_r4/White Gaussian  Noise Generator/Box-Muller4/fr1/lfsr_31_2/x6 ==
  " " : Inport  OutDataType=sfix(16)  OutScaling=2^0
  reset : Inport  Port=2  OutDataType=sfix(16)  OutScaling=2^0
  ASR : Subsystem  mask{init=[init(6) init(5) init(4) init(3) init(2) init(1)]}
      mask prompts: init "Initial Value"
      mask init:
      | init_size = size(init);
      | asr_length = init_size(2);
  Register : xbsIndex_r4/Register  init=init(7)  rst=on  en=off  dbl_ovrd=off  block_type=register
      settings: xl_area=[0, 0, 0, 0, 0, 0, 0]  block_version=VER_STRING_GOES_HERE
  z-7 : Outport  OutDataType=sfix(16)  OutScaling=2^0
  wires:
  Register/1 -> ASR/1(din)
  " "/1 -> Register/1
  ASR/1(dout) -> z-7/1
  reset/1 -> Register/2

== system xrbsComm_r4/White Gaussian  Noise Generator/Box-Muller4/fr1/lfsr_31_2/x7 ==
  " " : Inport  OutDataType=sfix(16)  OutScaling=2^0
  reset : Inport  Port=2  OutDataType=sfix(16)  OutScaling=2^0
  ASR : Subsystem  mask{init=[init(6) init(5) init(4) init(3) init(2) init(1)]}
      mask prompts: init "Initial Value"
      mask init:
      | init_size = size(init);
      | asr_length = init_size(2);
  Register : xbsIndex_r4/Register  init=init(7)  rst=on  en=off  dbl_ovrd=off  block_type=register
      settings: xl_area=[0, 0, 0, 0, 0, 0, 0]  block_version=VER_STRING_GOES_HERE
  z-7 : Outport  OutDataType=sfix(16)  OutScaling=2^0
  wires:
  Register/1 -> ASR/1(din)
  ASR/1(dout) -> z-7/1
  " "/1 -> Register/1
  reset/1 -> Register/2

== system xrbsComm_r4/White Gaussian  Noise Generator/Box-Muller4/fr1/lfsr_31_2/x8 ==
  " " : Inport  OutDataType=sfix(16)  OutScaling=2^0
  reset : Inport  Port=2  OutDataType=sfix(16)  OutScaling=2^0
  ASR : Subsystem  mask{init=[init(5) init(4) init(3) init(2) init(1)]}
      mask prompts: init "Initial Value"
      mask init:
      | init_size = size(init);
      | asr_length = init_size(2);
  Register : xbsIndex_r4/Register  init=init(6)  rst=on  en=off  dbl_ovrd=off  block_type=register
      settings: xl_area=[0, 0, 0, 0, 0, 0, 0]  block_version=VER_STRING_GOES_HERE
  z-6 : Outport  OutDataType=sfix(16)  OutScaling=2^0
  wires:
  Register/1 -> ASR/1(din)
  " "/1 -> Register/1
  ASR/1(dout) -> z-6/1
  reset/1 -> Register/2

== system xrbsComm_r4/White Gaussian  Noise Generator/Box-Muller4/fr1/lfsr_41_2/x1 ==
  " " : Inport  OutDataType=sfix(16)  OutScaling=2^0
  reset : Inport  Port=2  OutDataType=sfix(16)  OutScaling=2^0
  ASR : Subsystem  mask{init=[init(8) init(7) init(6) init(5) init(4) init(3) init(2) init(1)]}
      mask prompts: init "Initial Value"
      mask init:
      | init_size = size(init);
      | asr_length = init_size(2);
  Register1 : xbsIndex_r4/Register  init=init(9)  rst=on  en=off  dbl_ovrd=off  block_type=register
      settings: xl_area=[0, 0, 0, 0, 0, 0, 0]  block_version=VER_STRING_GOES_HERE
  z-9 : Outport  OutDataType=sfix(16)  OutScaling=2^0
  wires:
  ASR/1(dout) -> z-9/1
  " "/1 -> Register1/1
  Register1/1 -> ASR/1(din)
  reset/1 -> Register1/2

== system xrbsComm_r4/White Gaussian  Noise Generator/Box-Muller4/fr1/lfsr_41_2/x5 ==
  " " : Inport  OutDataType=sfix(16)  OutScaling=2^0
  reset : Inport  Port=2  OutDataType=sfix(16)  OutScaling=2^0
  ASR : Subsystem  mask{init=[init(9) init(8) init(7) init(6) init(5) init(4) init(3) init(2) init(1)]}
      mask prompts: init "Initial Value"
      mask init:
      | init_size = size(init);
      | asr_length = init_size(2);
  Register : xbsIndex_r4/Register  init=init(10)  rst=on  en=off  dbl_ovrd=off  block_type=register
      settings: xl_area=[0, 0, 0, 0, 0, 0, 0]  block_version=VER_STRING_GOES_HERE
  z-10 : Outport  OutDataType=sfix(16)  OutScaling=2^0
  wires:
  Register/1 -> ASR/1(din)
  ASR/1(dout) -> z-10/1
  " "/1 -> Register/1
  reset/1 -> Register/2

== system xrbsComm_r4/White Gaussian  Noise Generator/Box-Muller4/fr1/lfsr_41_2/x6 ==
  " " : Inport  OutDataType=sfix(16)  OutScaling=2^0
  reset : Inport  Port=2  OutDataType=sfix(16)  OutScaling=2^0
  ASR : Subsystem  mask{init=[init(8) init(7) init(6) init(5) init(4) init(3) init(2) init(1)]}
      mask prompts: init "Initial Value"
      mask init:
      | init_size = size(init);
      | asr_length = init_size(2);
  Register1 : xbsIndex_r4/Register  init=init(9)  rst=on  en=off  dbl_ovrd=off  block_type=register
      settings: xl_area=[0, 0, 0, 0, 0, 0, 0]  block_version=VER_STRING_GOES_HERE
  z-9 : Outport  OutDataType=sfix(16)  OutScaling=2^0
  wires:
  ASR/1(dout) -> z-9/1
  " "/1 -> Register1/1
  Register1/1 -> ASR/1(din)
  reset/1 -> Register1/2

== system xrbsComm_r4/White Gaussian  Noise Generator/Box-Muller4/fr1/lfsr_41_2/x7 ==
  " " : Inport  OutDataType=sfix(16)  OutScaling=2^0
  reset : Inport  Port=2  OutDataType=sfix(16)  OutScaling=2^0
  ASR : Subsystem  mask{init=[init(8) init(7) init(6) init(5) init(4) init(3) init(2) init(1)]}
      mask prompts: init "Initial Value"
      mask init:
      | init_size = size(init);
      | asr_length = init_size(2);
  Register1 : xbsIndex_r4/Register  init=init(9)  rst=on  en=off  dbl_ovrd=off  block_type=register
      settings: xl_area=[0, 0, 0, 0, 0, 0, 0]  block_version=VER_STRING_GOES_HERE
  z-9 : Outport  OutDataType=sfix(16)  OutScaling=2^0
  wires:
  ASR/1(dout) -> z-9/1
  Register1/1 -> ASR/1(din)
  " "/1 -> Register1/1
  reset/1 -> Register1/2

== system xrbsComm_r4/White Gaussian  Noise Generator/Box-Muller4/g2/lfsr_47_5/x10 ==
  "  " : Inport  OutDataType=sfix(16)  OutScaling=2^0
  reset : Inport  Port=2  OutDataType=sfix(16)  OutScaling=2^0
  ASR : Subsystem  mask{init=[init(4) init(3) init(2) init(1)]}
      mask prompts: init "Initial Value"
      mask init:
      | init_size = size(init);
      | asr_length = init_size(2);
  Register5 : xbsIndex_r4/Register  init=init(5)  rst=on  en=off  dbl_ovrd=off  block_type=register
      settings: xl_area=[0, 0, 0, 0, 0, 0, 0]  block_version=VER_STRING_GOES_HERE
  z-5 : Outport  OutDataType=sfix(16)  OutScaling=2^0
  wires:
  ASR/1(dout) -> z-5/1
  Register5/1 -> ASR/1(din)
  "  "/1 -> Register5/1
  reset/1 -> Register5/2

== system xrbsComm_r4/White Gaussian  Noise Generator/Box-Muller4/g2/lfsr_47_5/x11 ==
  " " : Inport  OutDataType=sfix(16)  OutScaling=2^0
  reset : Inport  Port=2  OutDataType=sfix(16)  OutScaling=2^0
  ASR : Subsystem  mask{init=[init(4) init(3) init(2) init(1)]}
      mask prompts: init "Initial Value"
      mask init:
      | init_size = size(init);
      | asr_length = init_size(2);
  Register : xbsIndex_r4/Register  init=init(5)  rst=on  en=off  dbl_ovrd=off  block_type=register
      settings: xl_area=[0, 0, 0, 0, 0, 0, 0]  block_version=VER_STRING_GOES_HERE
  z-5 : Outport  OutDataType=sfix(16)  OutScaling=2^0
  wires:
  ASR/1(dout) -> z-5/1
  Register/1 -> ASR/1(din)
  " "/1 -> Register/1
  reset/1 -> Register/2

== system xrbsComm_r4/White Gaussian  Noise Generator/Box-Muller4/g2/lfsr_47_5/x12 ==
  " " : Inport  OutDataType=sfix(16)  OutScaling=2^0
  reset : Inport  Port=2  OutDataType=sfix(16)  OutScaling=2^0
  ASR : Subsystem  mask{init=[init(4) init(3) init(2) init(1)]}
      mask prompts: init "Initial Value"
      mask init:
      | init_size = size(init);
      | asr_length = init_size(2);
  Register : xbsIndex_r4/Register  init=init(5)  rst=on  en=off  dbl_ovrd=off  block_type=register
      settings: xl_area=[0, 0, 0, 0, 0, 0, 0]  block_version=VER_STRING_GOES_HERE
  z-5 : Outport  OutDataType=sfix(16)  OutScaling=2^0
  wires:
  ASR/1(dout) -> z-5/1
  Register/1 -> ASR/1(din)
  " "/1 -> Register/1
  reset/1 -> Register/2

== system xrbsComm_r4/White Gaussian  Noise Generator/Box-Muller4/g2/lfsr_47_5/x13 ==
  note: reset
  " " : Inport  OutDataType=sfix(16)  OutScaling=2^0
  " 1" : Inport  Port=2  OutDataType=sfix(16)  OutScaling=2^0
  ASR : Subsystem  mask{init=[init(4) init(3) init(2) init(1)]}
      mask prompts: init "Initial Value"
      mask init:
      | init_size = size(init);
      | asr_length = init_size(2);
  Register : xbsIndex_r4/Register  init=init(5)  rst=on  en=off  dbl_ovrd=off  block_type=register
      settings: xl_area=[0, 0, 0, 0, 0, 0, 0]  block_version=VER_STRING_GOES_HERE
  z-5 : Outport  OutDataType=sfix(16)  OutScaling=2^0
  wires:
  ASR/1(dout) -> z-5/1
  Register/1 -> ASR/1(din)
  " "/1 -> Register/1
  " 1"/1 -> Register/2

== system xrbsComm_r4/White Gaussian  Noise Generator/Box-Muller4/g2/lfsr_47_5/x14 ==
  " " : Inport  OutDataType=sfix(16)  OutScaling=2^0
  reset : Inport  Port=2  OutDataType=sfix(16)  OutScaling=2^0
  ASR : Subsystem  mask{init=[init(4) init(3) init(2) init(1)]}
      mask prompts: init "Initial Value"
      mask init:
      | init_size = size(init);
      | asr_length = init_size(2);
  Register : xbsIndex_r4/Register  init=init(5)  rst=on  en=off  dbl_ovrd=off  block_type=register
      settings: xl_area=[0, 0, 0, 0, 0, 0, 0]  block_version=VER_STRING_GOES_HERE
  z-5 : Outport  OutDataType=sfix(16)  OutScaling=2^0
  wires:
  ASR/1(dout) -> z-5/1
  Register/1 -> ASR/1(din)
  " "/1 -> Register/1
  reset/1 -> Register/2

== system xrbsComm_r4/White Gaussian  Noise Generator/Box-Muller4/g2/lfsr_47_5/x15 ==
  " " : Inport  OutDataType=sfix(16)  OutScaling=2^0
  reset : Inport  Port=2  OutDataType=sfix(16)  OutScaling=2^0
  ASR : Subsystem  mask{init=[init(4) init(3) init(2) init(1)]}
      mask prompts: init "Initial Value"
      mask init:
      | init_size = size(init);
      | asr_length = init_size(2);
  Register : xbsIndex_r4/Register  init=init(5)  rst=on  en=off  dbl_ovrd=off  block_type=register
      settings: xl_area=[0, 0, 0, 0, 0, 0, 0]  block_version=VER_STRING_GOES_HERE
  z-5 : Outport  OutDataType=sfix(16)  OutScaling=2^0
  wires:
  ASR/1(dout) -> z-5/1
  Register/1 -> ASR/1(din)
  " "/1 -> Register/1
  reset/1 -> Register/2

== system xrbsComm_r4/White Gaussian  Noise Generator/Box-Muller4/g2/lfsr_47_5/x16 ==
  " " : Inport  OutDataType=sfix(16)  OutScaling=2^0
  reset : Inport  Port=2  OutDataType=sfix(16)  OutScaling=2^0
  ASR : Subsystem  mask{init=[init(3) init(2) init(1)]}
      mask prompts: init "Initial Value"
      mask init:
      | init_size = size(init);
      | asr_length = init_size(2);
  Register : xbsIndex_r4/Register  init=init(4)  rst=on  en=off  dbl_ovrd=off  block_type=register
      settings: xl_area=[0, 0, 0, 0, 0, 0, 0]  block_version=VER_STRING_GOES_HERE
  z-4 : Outport  OutDataType=sfix(16)  OutScaling=2^0
  wires:
  ASR/1(dout) -> z-4/1
  Register/1 -> ASR/1(din)
  " "/1 -> Register/1
  reset/1 -> Register/2

== system xrbsComm_r4/White Gaussian  Noise Generator/Box-Muller4/g2/lfsr_47_5/x9 ==
  " " : Inport  OutDataType=sfix(16)  OutScaling=2^0
  reset : Inport  Port=2  OutDataType=sfix(16)  OutScaling=2^0
  ASR : Subsystem  mask{init=[init(4) init(3) init(2) init(1)]}
      mask prompts: init "Initial Value"
      mask init:
      | init_size = size(init);
      | asr_length = init_size(2);
  Register : xbsIndex_r4/Register  init=init(5)  rst=on  en=off  dbl_ovrd=off  block_type=register
      settings: xl_area=[0, 0, 0, 0, 0, 0, 0]  block_version=VER_STRING_GOES_HERE
  z-5 : Outport  OutDataType=sfix(16)  OutScaling=2^0
  wires:
  ASR/1(dout) -> z-5/1
  Register/1 -> ASR/1(din)
  " "/1 -> Register/1
  reset/1 -> Register/2
